simulink model "MPCdouble"  (R2023a)
settings: Solver=ode15s  StartTime=0.0  StopTime=0.6  RelTol=1e-3  EnableMultiTasking=on
InitFcn:
  | TSG=5e-5;
  | Pn=4;
  | Ts=1e-6
undefined symbols (not defined in the file): sigbuilder_block
libraries: spsDCVoltageSourceLib x1, simulink x1, powerlib_extras x1, slpidlib x1, spsPermanentMagnetSynchronousMachineLib x1, spsUniversalBridgeLib x1, spsVoltageMeasurementLib x1, spspowerguiLib x1
settings Model: Creator=Administrator  LastModifiedBy=26271
settings SolverCC: AlgebraicLoopSolver=TrustRegion
settings DataIOCC: ReturnWorkspaceOutputs=off
settings OptimizationCC: LifeSpan=inf
settings DebuggingCC: UnconnectedInputMsg=warning  UnconnectedOutputMsg=warning  UnconnectedLineMsg=warning  SFUnexpectedBacktrackingDiag=warning  SFNoUnconditionalDefaultTransitionDiag=warning  ArithmeticOperatorsInVariantConditions=warning
settings ModelReferenceCC: EnableRefExpFcnMdlSchedulingChecks=on
settings SFSimCC: SimUseLocalCustomCode=off  CustomCodeUndefinedFunction=UseInterfaceOnly
settings RTWCC: RTWUseLocalCustomCode=off  DLArmComputeVersion=19.05
settings CodeAppCC: StateflowObjectComments=on
settings GRTTargetCC: TargetLangStandard=C89/C90 (ANSI)
settings ConfigComp: CovMetricSettings=dw  CovSaveCumulativeToWorkspaceVar=on  CovSaveSingleToWorkspaceVar=on  CovExternalEMLEnable=off
settings SimscapeCC: SimscapeNormalizeSystem=off

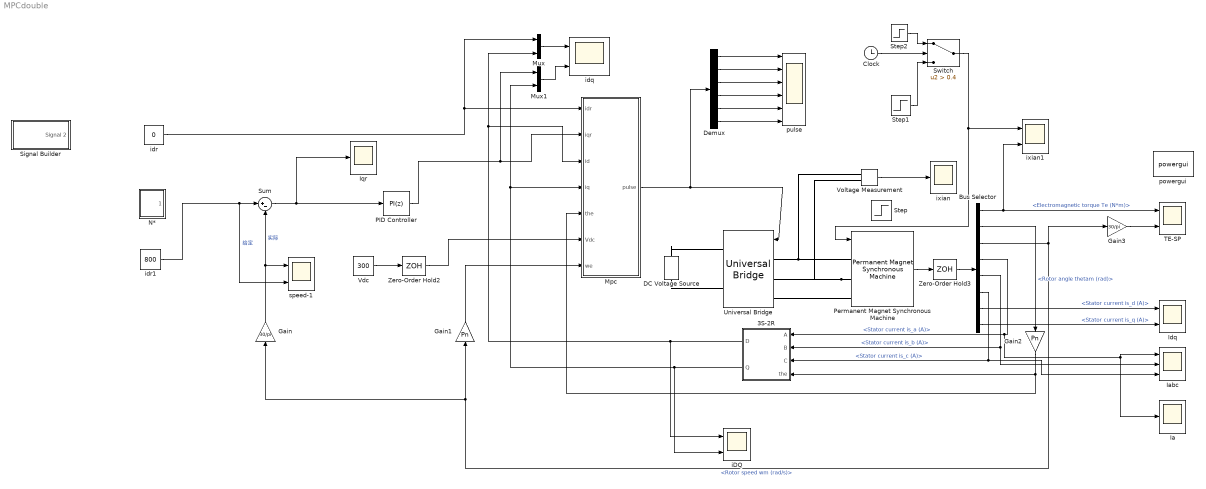
== system MPCdouble ==
  3S-2R : Subsystem
  Bus Selector : BusSelector  OutputSignals=Electromagnetic torque Te (N*m),Rotor angle thetam (rad),Rotor speed wm (rad/s),Stator current is_a (A),Stator current is_b (A),Stator current is_c (A),Stator current is_d (A),Stator current is_q (A)
  Clock : Clock
  DC Voltage Source : spsDCVoltageSourceLib/DC Voltage Source  Amplitude=300  Measurements=None
  Demux : Demux  Outputs=6
  Gain : Gain  Gain=30/pi
  Gain1 : Gain  Gain=Pn
  Gain2 : Gain  Gain=Pn
  Gain3 : Gain  Gain=30/pi
  Ia : Scope
  Iabc : Scope  NumInputPorts=3
  Idq : Scope  NumInputPorts=2
  Iqr : Scope
  Mpc : Subsystem
  Mux : Mux  Inputs=2
  Mux1 : Mux  Inputs=2
  N* : Subsystem
  PID Controller : slpidlib/PID Controller  Controller=PI  Form=Parallel  TimeDomain=Discrete-time  UseExternalTs=off  SampleTime=TSG  IntegratorMethod=Forward Euler  FilterMethod=Forward Euler  ControllerParametersSource=internal  P=0.18  I=16  UseKiTs=off  D=0  N=100  UseFilter=on  TunerSelectOption=Transfer Function Based (PID Tuner App)  InitialConditionSource=internal  InitialConditionForIntegrator=0  InitialConditionForFilter=0  DifferentiatorICPrevScaledInput=0  ExternalReset=none  TrackingMode=off  Kt=1  LimitOutput=on  SatLimitsSource=internal  UpperSaturationLimit=8  LowerSaturationLimit=-8  LinearizeAsGain=on  AntiWindupMode=none  Kb=1  LimitIntegrator=off  UpperIntegratorSaturationLimit=inf  LowerIntegratorSaturationLimit=-inf  POutMin=[]  POutMax=[]  IOutMin=[]  IOutMax=[]  DOutMin=[]  DOutMax=[]  NOutMin=[]  NOutMax=[]  SumOutMin=[]  SumOutMax=[]  SaturationOutMin=[]  SaturationOutMax=[]  PParamMin=[]  PParamMax=[]  IParamMin=[]  IParamMax=[]  DParamMin=[]  DParamMax=[]  NParamMin=[]  NParamMax=[]  KbParamMin=[]  KbParamMax=[]  KtParamMin=[]  KtParamMax=[]  KbOutMin=[]  KbOutMax=[]  KtOutMin=[]  KtOutMax=[]  IntegratorOutMin=[]  IntegratorOutMax=[]  FilterOutMin=[]  FilterOutMax=[]  SumI1OutMin=[]  SumI1OutMax=[]  SumI2OutMin=[]  SumI2OutMax=[]  SumI3OutMin=[]  SumI3OutMax=[]  SumI4OutMin=[]  SumI4OutMax=[]  SumDOutMin=[]  SumDOutMax=[]  DifferentiatorOutMin=[]  DifferentiatorOutMax=[]  FilterDiffOutCoefMin=[]  FilterDiffOutCoefMax=[]  ReciprocalOutMin=[]  ReciprocalOutMax=[]  SumDenOutMin=[]  SumDenOutMax=[]  SumNumOutMin=[]  SumNumOutMax=[]  DivideOutMin=[]  DivideOutMax=[]  UdiffTsProdOutMin=[]  UdiffTsProdOutMax=[]  NTsProdOutMin=[]  NTsProdOutMax=[]  UintegralTsProdOutMin=[]  UintegralTsProdOutMax=[]  UngainTsProdOutMin=[]  UngainTsProdOutMax=[]  ClampingZeroOutDataTypeStr=Inherit: Inherit via back propagation  ClampingZeroOutMin=[]  ClampingZeroOutMax=[]  FilterDenConstantOutDataTypeStr=Inherit: Inherit via back propagation  FilterDenConstantOutMin=[]  FilterDenConstantOutMax=[]  PCopyOutDataTypeStr=Inherit: Inherit via back propagation  PCopyOutMin=[]  PCopyOutMax=[]  NCopyOutDataTypeStr=Inherit: Inherit via back propagation  NCopyOutMin=[]  NCopyOutMax=[]  IntegratorContinuousStateAttributes=''  IntegratorStateMustResolveToSignalObject=off  IntegratorRTWStateStorageClass=Auto  FilterContinuousStateAttributes=''  FilterStateMustResolveToSignalObject=off  FilterRTWStateStorageClass=Auto  ParallelPVariant=InternalParameters  IdealPVariant=Disabled  IVariant=InternalParameters  DVariant=Disabled  IntegratorVariant=Discrete  SatVariant=Enabled  AWVariant=Passthrough  PCopyVariant=Disabled  TRVariant=Disabled  FdbkBlocksVariant=Forward  IdealPFdbkVariant=Disabled  SatFdbkVariant=Disabled  DerivativeFilterVariant=Disabled  NVariant=Disabled  NCopyVariant=Disabled_SignalSpec  FilterICVariant=Disabled  IntegratorICVariant=InternalICs  ExternalResetVariant=Disabled  TRSumVariant=Passthrough  SumFdbkVariant=Disabled  SumVariant=Sum_PI  TsampFilterVariant=InternalTs  TsampNgainVariant=Passthrough  TsampIntegralVariant=Disabled_SignalSpec  ExternalSaturationOutDataTypeStr=Inherit: Same as second input
  Permanent Magnet Synchronous Machine : spsPermanentMagnetSynchronousMachineLib/Permanent Magnet Synchronous Machine  NbPhases=3  FluxDistribution=Sinusoidal  RotorType=Round  MechanicalLoad=Torque Tm  PresetModel="05:  8 Nm 300 Vdc 2000 RPM - 10 Nm"  ShowDetailedParameters=on  MeasurementBus=off  Resistance=0.9585  Inductance=8.5e-3  dqInductances=[8.5e-3,8.5e-3]  La=0.00525  MachineConstant=Flux linkage established by magnets (V.s)  Flux=0.1827  VoltageCst=132.5525  TorqueCst=1.0962  Flat=120  Mechanical=[0.0006329 0.0003035 4 0]  PolePairs=4  InitialConditions=[0,0, 0,0]  InitialConditions5ph=[0 0 0 0 0 0]  RefAngle=Aligned with phase A axis (original Park)  IterativeDiscreteModel=Trapezoidal non iterative  TsBlock=-1  TsPowergui=0
  Signal Builder : Subsystem  Tag=STV Subsys  LoadFcn=sigbuilder_block('load');  StartFcn=sigbuilder_block('start');  StopFcn=sigbuilder_block('stop');  ClipboardFcn=sigbuilder_block('clipboard');  mask(Sigbuilder block){tuvar=[0:10]}
      mask help: Simulink:masks:SigbuilderBlock_MD
      mask init:
      | if ~strcmp(get_param(bdroot(gcbh),'SimulationStatus'),'stopped') tuvar = sigbuilder_block('maskInit'); end
      settings: CopyFcn=sigbuilder_block('copy');  DeleteFcn=sigbuilder_block('delete');  ModelCloseFcn=sigbuilder_block('modelClose');  PreSaveFcn=sigbuilder_block('preSave');  PauseFcn=sigbuilder_block('pause');  ContinueFcn=sigbuilder_block('continue');  NameChangeFcn=sigbuilder_block('namechange');  OpenFcn=sigbuilder_block('open',[437.6 199.2 550.4 400 ]);  CloseFcn=sigbuilder_block('close');
      mask Display: plot(0, 0, 100, 100,[2, 2, 32, 32, 2], [68, 8, 8, 68, 68],[32, 2], [38, 38], [32, 19, 2],[53, 60, 44], [32, 17, 17, 2],[16, 16, 31, 31]);txt = getActiveGroup(gcbh);text(2, 100, txt,'verticalAlignment', 'top');
  Step : Step  Time=0  After=5  SampleTime=0
  Step1 : Step  Time=0.2  After=2  SampleTime=0
  Step2 : Step  Time=0  After=5  SampleTime=0
  Sum : Sum  Inputs=|+-
  Switch : Switch  Criteria=u2 > Threshold  Threshold=0.4  ZeroCross=off  SaturateOnIntegerOverflow=off  InputSameDT=off
  TE-SP : Scope  NumInputPorts=2
  Universal Bridge : spsUniversalBridgeLib/Universal Bridge  Arms=3  SnubberResistance=1e5  SnubberCapacitance=inf  Device=IGBT / Diodes  Ron=1e-3  Lon=0  ForwardVoltages="[  0  0  ]"  ForwardVoltage=0  GTOparameters=[ 10e-6 , 20e-6 ]  IGBTparameters=[ 1e-6 , 2e-6 ]  Measurements=None  Measurements_2=None  converterType=Rectifier
  Vdc : Constant  Value=300
  Voltage Measurement : spsVoltageMeasurementLib/Voltage Measurement  PhasorSimulation=off  OutputType=Complex  PSBequivalent=0
  Zero-Order Hold2 : ZeroOrderHold  SampleTime=TSG
  Zero-Order Hold3 : ZeroOrderHold  SampleTime=TSG
  iDQ : Scope  NumInputPorts=2
  idq : Scope  NumInputPorts=2
  idr : Constant  Value=0
  idr1 : Constant  Value=800
  ixian : Scope
  ixian1 : Scope  NumInputPorts=2
  powergui : spspowerguiLib/powergui  Priority=1  SimulationMode=Discrete  SampleTime=Ts  frequency=60  Iterations=50  frequencyindice=0  Pbase=100e6  ErrMax=1e-4  UnitsV=kV  UnitsW=MW  buscounter=0  FunctionMessages=off  echomessages=off  EnableUseOfTLC=off  CurrentSourceSwitches=off  DisableSnubberDevices=off  DisableRonSwitches=off  DisableVfSwitches=off  DisplayEquations=off  AutomaticDiscreteSolvers=off  SolverType=Tustin/Backward Euler (TBE)  Interpol=off  ExternalGateDelay=off  methode=off  Ts=10  x0status=blocks  SPID=off  SwTol=0  HookPort=off  NonlinearTolerance=1e-4  nMaxIteration=100  ContinueOnMaxIteration=off  RestoreLinks=warning  ResistiveCurrentMeasurement=off  Frange=[0:2:500]  Ylog=off  Xlog=on  ShowGrid=off  save=off  variable=ZData  structure=Ia  ZoomFFT=off  StartTime=0.7  cycles=1  DisplayStyle=1  fundamental=66.667  FreqAxis=off  MaxFrequency=11000  frequencyindicesteady=1  RmsSteady=1  display=off
  pulse : Scope  NumInputPorts=6
  speed-1 : Scope  NumInputPorts=2
  wires:
  Gain/1 -> speed-1/1, Sum/2  "实际"
  Gain1/1 -> Mpc/7(we)
  Vdc/1 -> Zero-Order Hold2/1
  Bus Selector/2 -> Gain2/1  "<Rotor angle thetam (rad)>"
  Bus Selector/3 -> Gain/1, Gain1/1, Gain3/1  "<Rotor speed wm (rad/s)>"
  Bus Selector/4 -> 3S-2R/1(A), Iabc/1, Ia/1  "<Stator current is_a (A)>"
  Bus Selector/5 -> Iabc/2, 3S-2R/2(B)  "<Stator current is_b (A)>"
  Bus Selector/6 -> Iabc/3, 3S-2R/3(C)  "<Stator current is_c (A)>"
  idr/1 -> Mpc/1(idr), Mux/1
  Zero-Order Hold2/1 -> Mpc/6(Vdc)
  Mux/1 -> idq/1
  Mux1/1 -> idq/2
  Bus Selector/7 -> Idq/1  "<Stator current is_d (A)>"
  Bus Selector/8 -> Idq/2  "<Stator current is_q (A)>"
  Bus Selector/1 -> ixian1/2, TE-SP/1  "<Electromagnetic torque Te (N*m)>"
  Gain3/1 -> TE-SP/2
  Mpc/1(pulse) -> Demux/1, Universal Bridge/1
  Voltage Measurement/1 -> ixian/1
  Demux/1 -> pulse/1
  Demux/2 -> pulse/2
  Demux/3 -> pulse/3
  Demux/4 -> pulse/4
  Demux/5 -> pulse/5
  Demux/6 -> pulse/6
  Sum/1 -> PID Controller/1, Iqr/1
  idr1/1 -> speed-1/2, Sum/1  "给定"
  PID Controller/1 -> Mpc/2(iqr), Mux1/1
  3S-2R/1(D) -> Mpc/3(id), Mux/2, iDQ/1
  3S-2R/2(Q) -> Mpc/4(iq), Mux1/2, iDQ/2
  Gain2/1 -> Mpc/5(the), 3S-2R/4(the)
  Permanent Magnet Synchronous Machine/1 -> Zero-Order Hold3/1
  Zero-Order Hold3/1 -> Bus Selector/1
  Step2/1 -> Switch/1
  Step1/1 -> Switch/3
  Clock/1 -> Switch/2
  Switch/1 -> Permanent Magnet Synchronous Machine/1, ixian1/1
  connections:
  Voltage Measurement/LConn1 -- Universal Bridge/LConn1 -- Permanent Magnet Synchronous Machine/LConn1
  Permanent Magnet Synchronous Machine/LConn2 -- Universal Bridge/LConn2 -- Voltage Measurement/LConn2
  DC Voltage Source/RConn1 -- Universal Bridge/RConn1
  Universal Bridge/LConn3 -- Permanent Magnet Synchronous Machine/LConn3
  DC Voltage Source/LConn1 -- Universal Bridge/RConn2

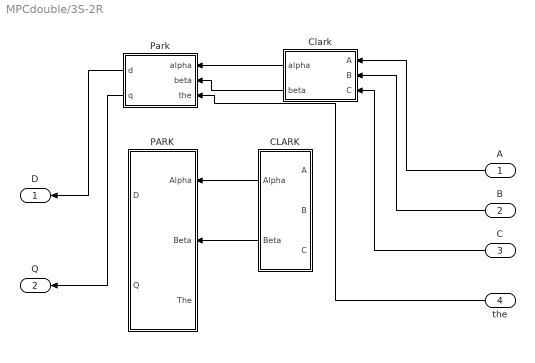
== system MPCdouble/3S-2R ==
  A : Inport
  B : Inport  Port=2
  C : Inport  Port=3
  the : Inport  Port=4
  CLARK : Subsystem
  Clark : MATLAB Function  TreatAsAtomicUnit=on
  PARK : Subsystem
  Park : MATLAB Function  TreatAsAtomicUnit=on
  D : Outport
  Q : Outport  Port=2
  wires:
  C/1 -> Clark/3(C)
  CLARK/1(Alpha) -> PARK/1(Alpha)
  A/1 -> Clark/1(A)
  CLARK/2(Beta) -> PARK/2(Beta)
  the/1 -> Park/3(the)
  B/1 -> Clark/2(B)
  Clark/1(alpha) -> Park/1(alpha)
  Clark/2(beta) -> Park/2(beta)
  Park/1(d) -> D/1
  Park/2(q) -> Q/1

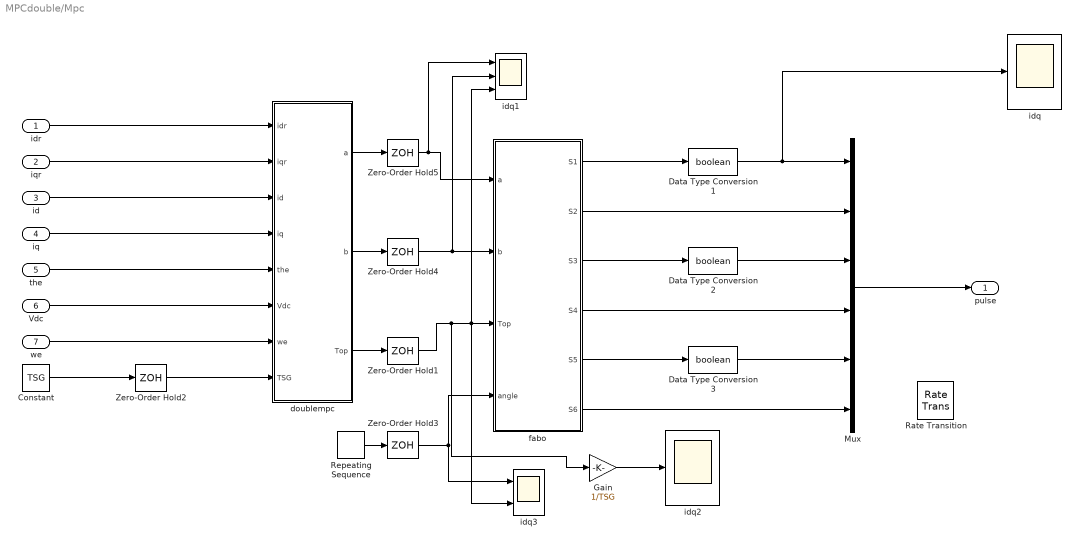
== system MPCdouble/Mpc ==
  idr : Inport
  iqr : Inport  Port=2
  id : Inport  Port=3
  iq : Inport  Port=4
  the : Inport  Port=5
  Vdc : Inport  Port=6
  we : Inport  Port=7
  Constant : Constant  Value=TSG
  Data Type Conversion1 : DataTypeConversion  OutDataTypeStr=boolean  SaturateOnIntegerOverflow=off  RndMeth=Floor
  Data Type Conversion2 : DataTypeConversion  OutDataTypeStr=boolean  SaturateOnIntegerOverflow=off  RndMeth=Floor
  Data Type Conversion3 : DataTypeConversion  OutDataTypeStr=boolean  SaturateOnIntegerOverflow=off  RndMeth=Floor
  Gain : Gain  Gain=1/TSG
  Mux : Mux  Inputs=6
  Rate Transition : RateTransition
  Repeating Sequence : simulink/Sources/Repeating Sequence  rep_seq_t=[0 TSG/2 TSG]  rep_seq_y=[0 TSG 0]
  Zero-Order Hold{1,3..5} (4 alike) : ZeroOrderHold  SampleTime=Ts
  Zero-Order Hold2 : ZeroOrderHold  SampleTime=TSG
  doublempc : MATLAB Function  TreatAsAtomicUnit=on
  fabo : MATLAB Function  TreatAsAtomicUnit=on
  idq : Scope
  idq1 : Scope  NumInputPorts=3
  idq2 : Scope
  idq3 : Scope  NumInputPorts=2
  pulse : Outport
  wires:
  Mux/1 -> pulse/1
  fabo/1(S1) -> Data Type Conversion1/1
  fabo/3(S3) -> Data Type Conversion2/1
  fabo/2(S2) -> Mux/2
  fabo/4(S4) -> Mux/4
  Data Type Conversion1/1 -> Mux/1, idq/1
  Data Type Conversion2/1 -> Mux/3
  Data Type Conversion3/1 -> Mux/5
  Constant/1 -> Zero-Order Hold2/1
  Zero-Order Hold2/1 -> doublempc/8(TSG)
  idr/1 -> doublempc/1(idr)
  iqr/1 -> doublempc/2(iqr)
  id/1 -> doublempc/3(id)
  iq/1 -> doublempc/4(iq)
  the/1 -> doublempc/5(the)
  Vdc/1 -> doublempc/6(Vdc)
  we/1 -> doublempc/7(we)
  fabo/5(S5) -> Data Type Conversion3/1
  fabo/6(S6) -> Mux/6
  Repeating Sequence/1 -> Zero-Order Hold3/1
  Zero-Order Hold3/1 -> idq3/1, fabo/4(angle)
  doublempc/1(a) -> Zero-Order Hold5/1
  doublempc/2(b) -> Zero-Order Hold4/1
  doublempc/3(Top) -> Zero-Order Hold1/1
  Zero-Order Hold1/1 -> Gain/1, idq3/2, fabo/3(Top), idq1/3
  Zero-Order Hold4/1 -> fabo/2(b), idq1/2
  Zero-Order Hold5/1 -> idq1/1, fabo/1(a)
  Gain/1 -> idq2/1

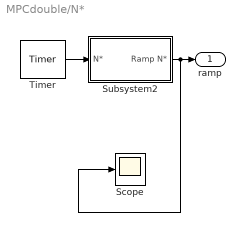
== system MPCdouble/N* ==
  Scope : Scope
  Subsystem2 : Subsystem
  Timer : powerlib_extras/Control  Blocks/Timer  t=[0 1]  e=[2000 2000]
  ramp : Outport
  wires:
  Timer/1 -> Subsystem2/1(N*)
  Subsystem2/1(Ramp N*) -> Scope/1, ramp/1

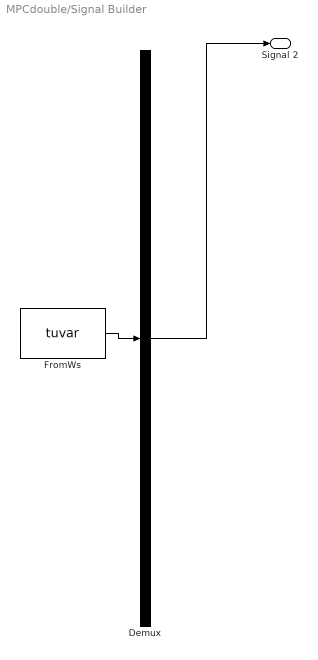
== system MPCdouble/Signal Builder ==
  Demux : Demux  Tag=STV Demux  Outputs=1
      settings: DisplayOption=none
  FromWs : FromWorkspace  Tag=STV FromWs  VariableName=tuvar
      SigBuilderData=|
      | common.afterFinalStr = 'Extrapolate'
      | common.sampleTime = 0
      | dataSet(1).timeRange = [0 0.6]
      | dataSet(1).name = 'Group 1'
      | dataSet(2).timeRange = [0 0.6]
      | dataSet(2).name = 'Group 2'
      | sbobj.Groups(1).Name = 'Group 1'
      | sbobj.Groups(1).Signals.Name = 'Signal 2'
      | sbobj.Groups(1).Signals.XData = [0 0.05 0.2 0.25 0.4 0.6]
      | sbobj.Groups(1).Signals.YData = [0 400 400 600 600 800]
      | sbobj.Groups(1).TimeRange = [0 0.6]
      | sbobj.Groups(2).Name = 'Group 2'
      | sbobj.Groups(2).Signals.Name = 'Signal 2'
      | sbobj.Groups(2).Signals.XData = [0 0.05 0.2 0.25 0.4 0.45 0.6]
      | sbobj.Groups(2).Signals.YData = [0 400 400 600 600 800 800]
      | sbobj.Groups(2).TimeRange = [0 0.6]
  Signal 2 : Outport  Tag=STV Outport
  wires:
  FromWs/1 -> Demux/1
  Demux/1 -> Signal 2/1

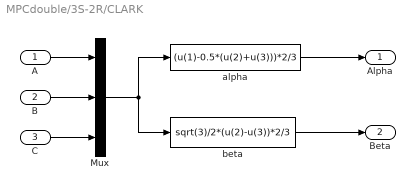
== system MPCdouble/3S-2R/CLARK ==
  A : Inport
  B : Inport  Port=2
  C : Inport  Port=3
  Mux : Mux  Inputs=3
  alpha : Fcn  Expr=(u(1)-0.5*(u(2)+u(3)))*2/3
  beta : Fcn  Expr=sqrt(3)/2*(u(2)-u(3))*2/3
  Alpha : Outport
  Beta : Outport  Port=2
  wires:
  beta/1 -> Beta/1
  alpha/1 -> Alpha/1
  Mux/1 -> alpha/1, beta/1
  C/1 -> Mux/3
  B/1 -> Mux/2
  A/1 -> Mux/1

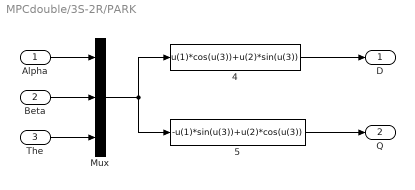
== system MPCdouble/3S-2R/PARK ==
  Alpha : Inport
  Beta : Inport  Port=2
  The : Inport  Port=3
  4 : Fcn  Expr=u(1)*cos(u(3))+u(2)*sin(u(3))
  5 : Fcn  Expr=-u(1)*sin(u(3))+u(2)*cos(u(3))
  Mux : Mux  Inputs=3
  D : Outport
  Q : Outport  Port=2
  wires:
  5/1 -> Q/1
  4/1 -> D/1
  Mux/1 -> 4/1, 5/1
  The/1 -> Mux/3
  Beta/1 -> Mux/2
  Alpha/1 -> Mux/1

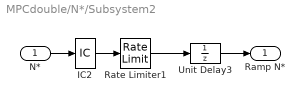
== system MPCdouble/N*/Subsystem2 ==
  N* : Inport
  IC2 : InitialCondition  Value=0
  Rate Limiter1 : RateLimiter  RisingSlewLimit=10000  FallingSlewLimit=-10000
  Unit Delay3 : UnitDelay  SampleTime=TSG  HasFrameUpgradeWarning=on
  Ramp N* : Outport
  wires:
  Unit Delay3/1 -> Ramp N*/1
  IC2/1 -> Rate Limiter1/1
  Rate Limiter1/1 -> Unit Delay3/1
  N*/1 -> IC2/1

== matlab function MPCdouble/3S-2R/Clark ==
  data: A input; B input; C input; alpha output; beta output
function [alpha,beta]=clark(A,B,C)
%#codegen
alpha=(A-0.5*(B+C))*2/3;
beta=sqrt(3)/2*(B-C)*2/3;
end

== matlab function MPCdouble/Mpc/fabo ==
  data: a input; S1 output; b input; Top input; angle input; S2 output; S3 output; S4 output; S5 output; S6 output
function [S1,S2,S3,S4,S5,S6]= fabo(a,b,Top,angle)

state=[0 0 0;1 0 0;1 1 0;0 1 0;0 1 1;0 0 1;1 0 1;0 0 0];

if angle<Top
S1=state(a,1); 
S3=state(a,2);
S5=state(a,3);
S2=~state(a,1);
S4=~state(a,2);
S6=~state(a,3);
else
S1=state(b,1); 
S3=state(b,2);
S5=state(b,3);
S2=~state(b,1);
S4=~state(b,2);
S6=~state(b,3);   
end

== matlab function MPCdouble/3S-2R/Park ==
  data: alpha input; beta input; d output; q output; the input
function [d,q]=park(alpha,beta,the)
%#codegen
d=alpha*cos(the)+beta*sin(the);
q=-alpha*sin(the)+beta*cos(the);
end

== matlab function MPCdouble/Mpc/doublempc ==
  data: idr input; iqr input; id input; iq input; the input; Vdc input; we input; TSG input; a output; b output; Top output
function [a,b,Top] = doublempc(idr,iqr,id,iq,the,Vdc,we,TSG)

persistent   e g Rs Ld Lq flux Vda Vqa Vdb Vqb a1 b2 T1 Topt


if isempty(Vda),Vda=0;  end
if isempty(Vqa),Vqa=0;  end
if isempty(Vdb),Vdb=0;  end
if isempty(Vqb),Vqb=0;  end
if isempty(a1),a1=0;    end
if isempty(b2),b2=0;    end
if isempty(T1),T1=TSG;  end
if isempty(Topt),Topt=TSG;  end

Rs=0.9585;
Ld=0.00525;
Lq=0.00525;
flux=0.1827;
e=1e10;
g=1e10;

%%%%%%%%%%%%%%%  电压矢量  %%%%%%%%%%%%%%%%%%%%
V0=0;
V1=2/3*Vdc;
V2=1/3*Vdc+1j*1/sqrt(3)*Vdc;
V3=-1/3*Vdc+1j*1/sqrt(3)*Vdc;
V4=-2/3*Vdc;
V5=-1/3*Vdc-1j*1/sqrt(3)*Vdc;
V6=1/3*Vdc-1j*1/sqrt(3)*Vdc;
V7=0;
V=[V0 V1 V2 V3 V4 V5 V6 V7];
% state=[0 0 0;1 0 0;1 1 0;0 1 0;0 1 1;0 0 1;1 0 1;0 0 0];

%%%%%%%%%%%%  枚举选择第一个最优电压矢量  %%%%%%%%%%%%%%%
for i=2:7
    Vo=V(i);
    Vd1=real(Vo)*cos(the)+imag(Vo)*sin(the);
    Vq1=-real(Vo)*sin(the)+imag(Vo)*cos(the);
    
    idk_1=(1-TSG*Rs/Ld)*id+we*TSG*Lq/Ld*iq+TSG/Ld*Vd1;
    iqk_1=(1-TSG*Rs/Lq)*iq-we*TSG*Ld/Lq*id+TSG/Ld*Vq1-we*flux*TSG/Lq;
 %%%%%%%%%%%%%%  一矢量价值函数  %%%%%%%%%%%%%%
    error=(idr-idk_1)^2+(iqr-iqk_1)^2;
    if error<e
        e=error;
        a1=i;
       Vda=Vd1;
       Vqa=Vq1;
    end 
end



%%%%%%%%%%%%  枚举选择第二个最优电压矢量  %%%%%%%%%%%%%%%
 for j=1:7
   Vj=V(j);
   k0=-Rs/Lq*iq-we*Ld/Lq*id-we*flux/Lq;     
   Vqq=-real(Vj)*sin(the)+imag(Vj)*cos(the); 
   kopt2=k0+Vqq/Lq;                          %第一个电压矢量作用时斜率
   kopt1=k0+Vqa/Lq;                          %第二个电压矢量作用时斜率
   Topt=(iqr-iq-kopt2*TSG)/(kopt1-kopt2);
   
   Vd_2=real(Vj)*cos(the)+imag(Vj)*sin(the);
   Vq_2=-real(Vj)*sin(the)+imag(Vj)*cos(the);
   
   Vd2=(Vda*Topt+Vd_2*(TSG-Topt))/TSG;      %合成电压
   Vq2=(Vqa*Topt+Vq_2*(TSG-Topt))/TSG;      %合成电压
   
   idk_2=(1-TSG*Rs/Ld)*id+we*TSG*Lq/Ld*iq+TSG/Ld*Vd2;
   iqk_2=(1-TSG*Rs/Lq)*iq-we*TSG*Ld/Lq*id+TSG/Ld*Vq2-we*flux*TSG/Lq;
   
%%%%%%%%%%%%%%  二矢量价值函数  %%%%%%%%%%%%%%
   gi=(idr-idk_2)^2+(iqr-iqk_2)^2;
    if gi<g
        g=gi;
        b2=j;
       Vdb=Vd2;
       Vqb=Vq2;
       T1=Topt;
    end 
 end
 
 if T1>TSG
     T1=TSG;
 elseif T1<0
     T1=0;
 end
 Top=T1;
 a=a1;
 b=b2;
end
